simulink model "Final_IMC_with_ADC"  (R2020a)
settings: Solver=ode14x  StartTime=0.0  StopTime=300  FixedStep=0.002  RelTol=1e-3
libraries: simulink x2
settings Model: Creator=therealtschmidt  LastModifiedBy=Noah

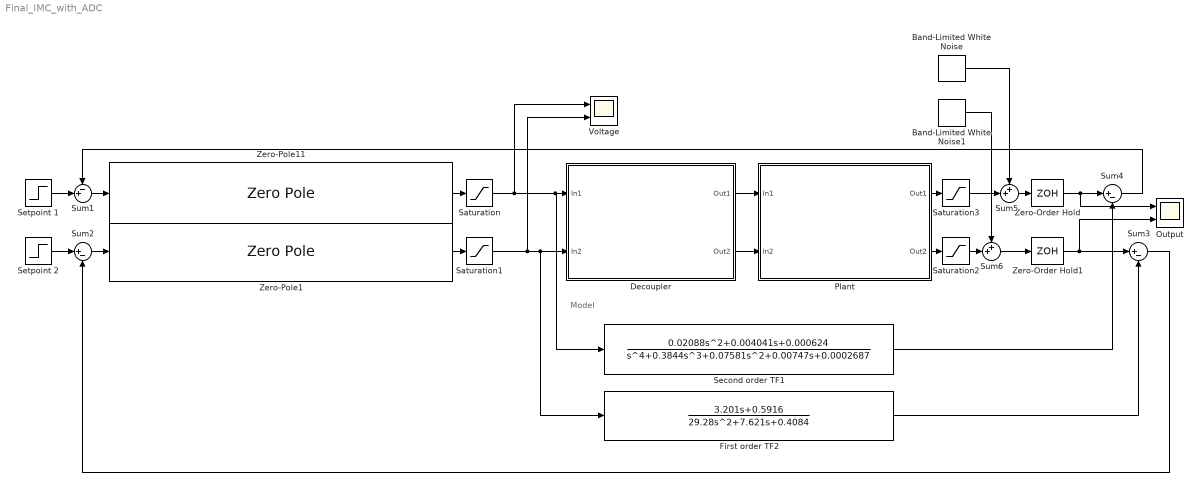
== system Final_IMC_with_ADC ==
  note: Model
  " Plant" : Subsystem
  Band-Limited White Noise : simulink/Sources/Band-Limited White Noise  Cov=0.001  Ts=0.1  seed=[23581]
  Band-Limited White Noise1 : simulink/Sources/Band-Limited White Noise  Cov=0.001  Ts=0.1  seed=[23341]
  Decoupler : Subsystem
  First order TF2 : TransferFcn  Numerator=[3.201 0.5916]  Denominator=[29.28 7.621 0.4084]
  Output : Scope  NumInputPorts=2
  Saturation : Saturate  UpperLimit=12  LowerLimit=0
  Saturation1 : Saturate  UpperLimit=12  LowerLimit=0
  Saturation2 : Saturate  UpperLimit=30  LowerLimit=0
  Saturation3 : Saturate  UpperLimit=30  LowerLimit=0
  Second order TF1 : TransferFcn  Numerator=[0.02088 0.004041 0.000624]  Denominator=[1 0.3844 0.07581 0.00747 0.0002687]
  Setpoint 1 : Step  Time=0  SampleTime=0
  Setpoint 2 : Step  Time=0  After=14  SampleTime=0
  Sum1 : Sum  Inputs=-+|
  Sum2 : Sum  Inputs=|+-
  Sum3 : Sum  Inputs=|+-
  Sum4 : Sum  Inputs=|+-
  Sum5 : Sum  Inputs=++|
  Sum6 : Sum  Inputs=++|
  Voltage : Scope  NumInputPorts=2
  Zero-Order Hold : ZeroOrderHold  SampleTime=0.002
  Zero-Order Hold1 : ZeroOrderHold  SampleTime=0.002
  Zero-Pole1 : ZeroPole  Zeros=[-0.1848 -0.0755]  Poles=[-0.1848 -0.10937]
  Zero-Pole11 : ZeroPole  Zeros=[-0.0961+0.1437i -0.0961-0.1437i -0.1116 -0.0806]  Poles=[-0.0961+0.1437i -0.0961-0.1437i -0.14455 -0.14455]
  wires:
  Decoupler/2(Out2) -> " Plant"/2(In2)
  Decoupler/1(Out1) -> " Plant"/1(In1)
  " Plant"/1(Out1) -> Saturation3/1
  Second order TF1/1 -> Sum4/2
  First order TF2/1 -> Sum3/2
  Saturation/1 -> Voltage/1, Second order TF1/1, Decoupler/1(In1)
  Saturation1/1 -> First order TF2/1, Decoupler/2(In2), Voltage/2
  Zero-Pole1/1 -> Saturation1/1
  Zero-Pole11/1 -> Saturation/1
  Band-Limited White Noise1/1 -> Sum6/1
  Band-Limited White Noise/1 -> Sum5/1
  Setpoint 2/1 -> Sum2/1
  Setpoint 1/1 -> Sum1/2
  Sum2/1 -> Zero-Pole1/1
  Sum1/1 -> Zero-Pole11/1
  Sum4/1 -> Sum1/1
  Sum3/1 -> Sum2/2
  Sum5/1 -> Zero-Order Hold/1
  Sum6/1 -> Zero-Order Hold1/1
  Zero-Order Hold/1 -> Output/1, Sum4/1
  Zero-Order Hold1/1 -> Output/2, Sum3/1
  Saturation2/1 -> Sum6/2
  " Plant"/2(Out2) -> Saturation2/1
  Saturation3/1 -> Sum5/2

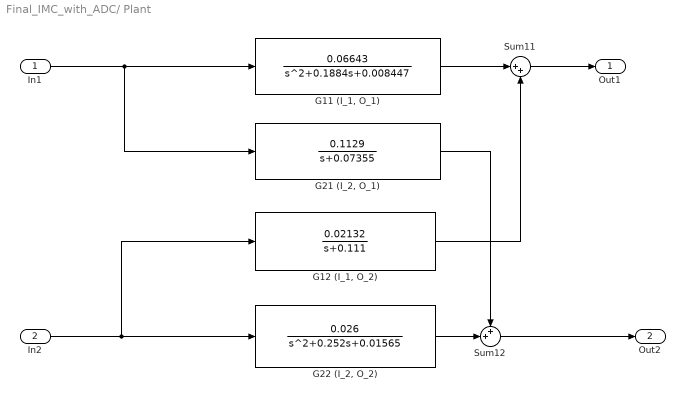
== system Final_IMC_with_ADC/ Plant ==
  In1 : Inport
  In2 : Inport  Port=2
  "G11 (I_1, O_1)" : TransferFcn  Numerator=0.06643  Denominator=[1 0.1884 0.008447]
  "G12 (I_1, O_2)" : TransferFcn  Numerator=0.02132  Denominator=[1 0.111]
  "G21 (I_2, O_1)" : TransferFcn  Numerator=0.1129  Denominator=[1 0.07355]
  "G22 (I_2, O_2)" : TransferFcn  Numerator=0.026  Denominator=[1 0.252 0.01565]
  Sum11 : Sum  Inputs=|++
  Sum12 : Sum  Inputs=++|
  Out1 : Outport  VectorParamsAs1DForOutWhenUnconnected=off
  Out2 : Outport  Port=2  VectorParamsAs1DForOutWhenUnconnected=off
  wires:
  "G22 (I_2, O_2)"/1 -> Sum12/2
  In1/1 -> "G11 (I_1, O_1)"/1, "G21 (I_2, O_1)"/1
  "G12 (I_1, O_2)"/1 -> Sum11/2
  "G11 (I_1, O_1)"/1 -> Sum11/1
  In2/1 -> "G12 (I_1, O_2)"/1, "G22 (I_2, O_2)"/1
  "G21 (I_2, O_1)"/1 -> Sum12/1
  Sum12/1 -> Out2/1
  Sum11/1 -> Out1/1

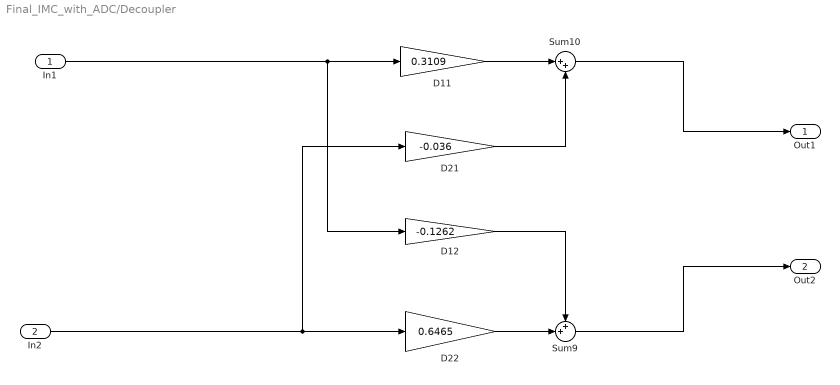
== system Final_IMC_with_ADC/Decoupler ==
  In1 : Inport
  In2 : Inport  Port=2
  D11 : Gain  Gain=0.3109
  D12 : Gain  Gain=-0.1262
  D21 : Gain  Gain=-0.036
  D22 : Gain  Gain=0.6465
  Sum10 : Sum  Inputs=|++
  Sum9 : Sum  Inputs=++|
  Out1 : Outport  VectorParamsAs1DForOutWhenUnconnected=off
  Out2 : Outport  Port=2  VectorParamsAs1DForOutWhenUnconnected=off
  wires:
  In1/1 -> D11/1, D12/1
  D12/1 -> Sum9/1
  D21/1 -> Sum10/2
  D22/1 -> Sum9/2
  In2/1 -> D21/1, D22/1
  Sum9/1 -> Out2/1
  D11/1 -> Sum10/1
  Sum10/1 -> Out1/1
